simulink model "untitled"  (R2022a)
settings: Solver=VariableStepAuto  StartTime=0.0  StopTime=10.0  RelTol=1e-3
values from neighbouring files (symbols this model uses):
  den = [2 1]    [class31323.m]
  Kd = 1    [class31323.m]
  Ki = 1    [class31323.m]
  Kp = 1    [class31323.m]
  num = [0.75]    [class31323.m]
settings Model: Creator=Estudiantes  LastModifiedBy=Estudiantes

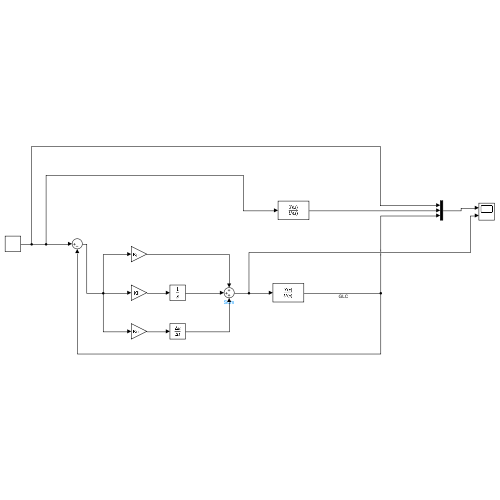
[thumbnail: Simulink's stored preview of the top-level diagram]
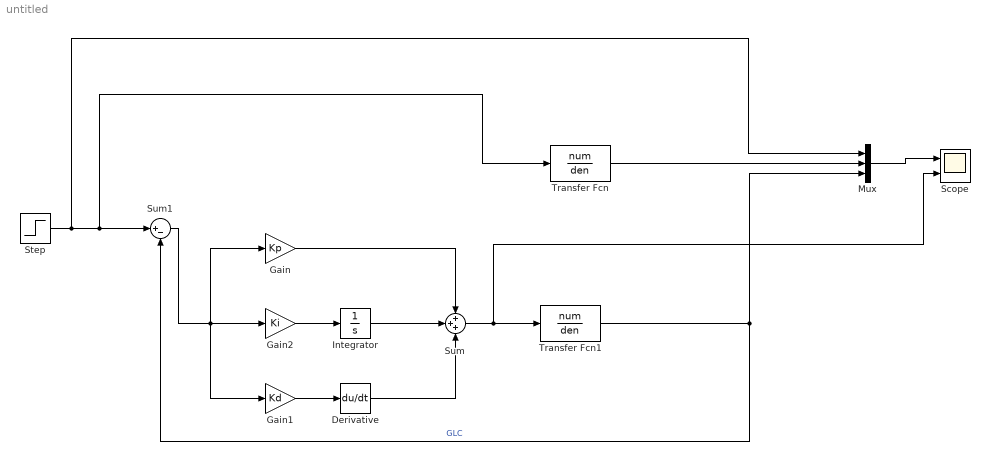
== system untitled ==
  Derivative : Derivative
  Gain : Gain  Gain=Kp
  Gain1 : Gain  Gain=Kd
  Gain2 : Gain  Gain=Ki
  Integrator : Integrator
  Mux : Mux  Inputs=3
  Scope : Scope  NumInputPorts=2
  Step : Step  Time=0  Before=1  SampleTime=0
  Sum : Sum  Inputs=+++
  Sum1 : Sum  Inputs=|+-
  Transfer Fcn : TransferFcn  Numerator=num  Denominator=den
  Transfer Fcn1 : TransferFcn  Numerator=num  Denominator=den
  wires:
  Gain2/1 -> Integrator/1
  Gain1/1 -> Derivative/1
  Gain/1 -> Sum/1
  Derivative/1 -> Sum/3
  Integrator/1 -> Sum/2
  Sum1/1 -> Gain1/1, Gain/1, Gain2/1
  Step/1 -> Mux/1, Transfer Fcn/1, Sum1/1
  Sum/1 -> Scope/2, Transfer Fcn1/1
  Transfer Fcn1/1 -> Mux/3, Sum1/2  "GLC"
  Mux/1 -> Scope/1
  Transfer Fcn/1 -> Mux/2
